simulink library "INT_InjCrv_PoI2Set"  (R2016b)
settings: Solver=VariableStepAuto  StartTime=0.0  StopTime=10.0  RelTol=1e-3
settings Model: Creator=Administrator  LastModifiedBy=Administrator

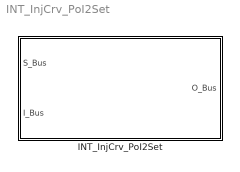
== system INT_InjCrv_PoI2Set ==
  INT_InjCrv_PoI2Set : Subsystem

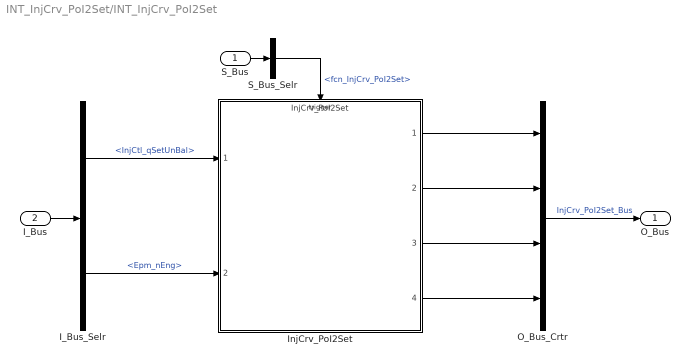
== system INT_InjCrv_PoI2Set/INT_InjCrv_PoI2Set ==
  S_Bus : Inport
  I_Bus : Inport  Port=2
  I_Bus_Selr : BusSelector  OutputSignals=InjCtl_qSetUnBal,Epm_nEng
  InjCrv_PoI2Set : ModelReference  ModelNameDialog=InjCrv_PoI2Set  SimulationMode=Normal  ModelReferenceVersion=1.5  TriggerPortName=function  TriggerPortTriggerType=function-call  TriggerPortStatesWhenEnabling=held
  O_Bus_Crtr : BusCreator  Inputs=4
  S_Bus_Selr : BusSelector  OutputSignals=fcn_InjCrv_PoI2Set
  O_Bus : Outport
  wires:
  S_Bus_Selr/1 -> InjCrv_PoI2Set/Trigger  "<fcn_InjCrv_PoI2Set>"
  S_Bus/1 -> S_Bus_Selr/1
  I_Bus/1 -> I_Bus_Selr/1
  I_Bus_Selr/1 -> InjCrv_PoI2Set/1  "<InjCtl_qSetUnBal>"
  I_Bus_Selr/2 -> InjCrv_PoI2Set/2  "<Epm_nEng>"
  O_Bus_Crtr/1 -> O_Bus/1  "InjCrv_PoI2Set_Bus"
  InjCrv_PoI2Set/1 -> O_Bus_Crtr/1
  InjCrv_PoI2Set/2 -> O_Bus_Crtr/2
  InjCrv_PoI2Set/3 -> O_Bus_Crtr/3
  InjCrv_PoI2Set/4 -> O_Bus_Crtr/4
